simulink model "dcmtrCtrl_PID_Harness0"  (R2021a)
settings: Solver=ode15s  StartTime=0.0  StopTime=25  RelTol=1e-3
libraries: simulink_extras x2
settings Model: DataDictionary=dcmtr_ctrl.sldd  Creator=smuckati  LastModifiedBy=smuckati
settings OptimizationCC: DefaultParameterBehavior=Inlined  UseDivisionForNetSlopeComputation=on  EnhancedBackFolding=on  PassReuseOutputArgsAs=Individual arguments  ZeroExternalMemoryAtStartup=off  ZeroInternalMemoryAtStartup=off  OptimizeBlockOrder=speed  DifferentSizesBufferReuse=on  OptimizationCustomize=off  EfficientTunableParamExpr=on
settings DebuggingCC: SignalRangeChecking=error  ParameterPrecisionLossMsg=none  ParameterTunabilityLossMsg=error
settings SFSimCC: MATLABDynamicMemAlloc=off
settings RTWCC: SystemTargetFile=ert.tlc  GenCodeOnly=on  TemplateMakefile=ert_default_tmf  CodeExecutionProfiling=on  CodeProfilingSaveOptions=AllData  CodeProfilingInstrumentation=detailed
settings CodeAppCC: ForceParamTrailComments=on  IgnoreCustomStorageClasses=off  OperatorAnnotations=on  SimulinkDataObjDesc=on  SFDataObjDesc=on  InsertBlockDesc=on
settings ERTTargetCC: TargetLangStandard=C99 (ISO)  GenerateSampleERTMain=on  InlinedParameterPlacement=NonHierarchical  ERTCustomFileTemplate=example_file_process.tlc

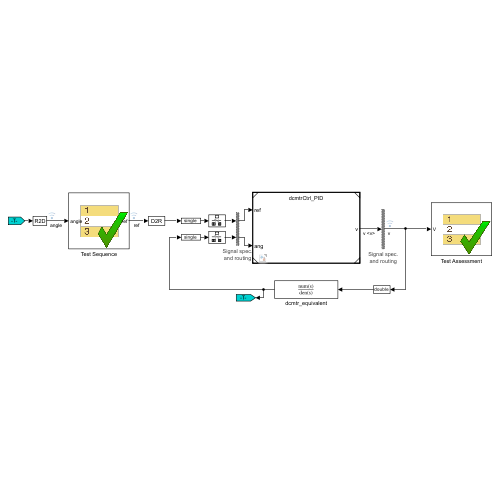
[thumbnail: Simulink's stored preview of the top-level diagram]
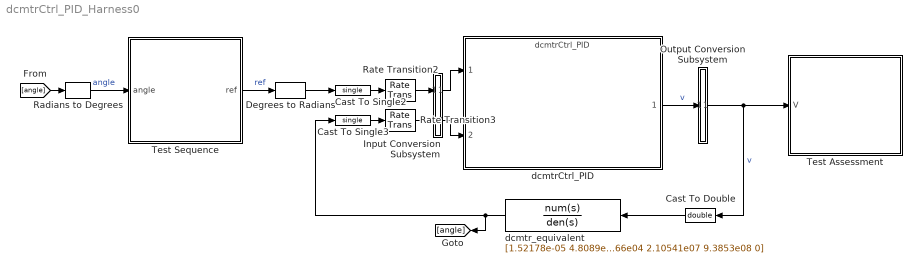
== system dcmtrCtrl_PID_Harness0 ==
  Cast To Double : DataTypeConversion  OutDataTypeStr=double
  Cast To Single2 : DataTypeConversion  OutDataTypeStr=single
  Cast To Single3 : DataTypeConversion  OutDataTypeStr=single
  Degrees to Radians : simulink_extras/Transformations/Degrees to Radians
  Input Conversion Subsystem : Subsystem  Tag=__SLT_ICS__  Description=|
      | Signal spec.
      | and routing
      settings: AttributesFormatString=%<Description>
  Output Conversion Subsystem : Subsystem  Tag=__SLT_OCS__  Description=|
      | Signal spec.
      | and routing
      settings: AttributesFormatString=%<Description>
  Radians to Degrees : simulink_extras/Transformations/Radians to Degrees
  Rate Transition2 : RateTransition  OutPortSampleTime=Ctrl_Ts
  Rate Transition3 : RateTransition  OutPortSampleTime=Ctrl_Ts
  Test Assessment : Test Sequence  TreatAsAtomicUnit=on
  Test Sequence : Test Sequence  TreatAsAtomicUnit=on
  dcmtrCtrl_PID : ModelReference  ModelNameDialog=dcmtrCtrl_PID  SimulationMode=Normal  ModelReferenceVersion=6.0
  dcmtr_equivalent : TransferFcn  Numerator=[1.52178e-05 4.8089e07]  Denominator=[1 1.74166e04 2.10541e07 9.3853e08 0]
  wires:
  Degrees to Radians/1 -> Cast To Single2/1
  Output Conversion Subsystem/1(Outport_1) -> Cast To Double/1, Test Assessment/1(V)  "v"
  Input Conversion Subsystem/1(Outport_1) -> dcmtrCtrl_PID/1
  Input Conversion Subsystem/2(Outport_2) -> dcmtrCtrl_PID/2
  dcmtrCtrl_PID/1 -> Output Conversion Subsystem/1(Inport_1)  "v"
  Cast To Single2/1 -> Rate Transition2/1
  Rate Transition2/1 -> Input Conversion Subsystem/1(Inport_1)
  Cast To Single3/1 -> Rate Transition3/1
  Rate Transition3/1 -> Input Conversion Subsystem/2(Inport_2)
  dcmtr_equivalent/1 -> [angle], Cast To Single3/1
  Cast To Double/1 -> dcmtr_equivalent/1
  Test Sequence/1(ref) -> Degrees to Radians/1  "ref"
  [angle] -> Radians to Degrees/1
  Radians to Degrees/1 -> Test Sequence/1(angle)  "angle"

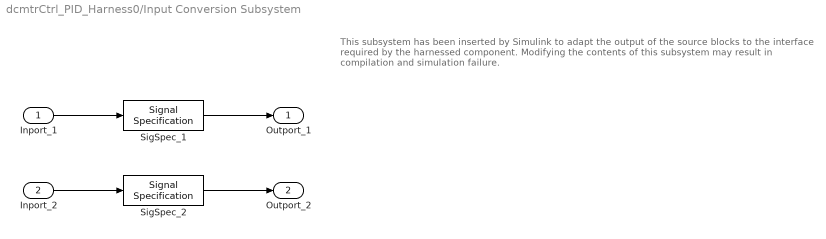
== system dcmtrCtrl_PID_Harness0/Input Conversion Subsystem ==
  note: This subsystem has been inserted by Simulink to adapt the output of the source blocks to the interface required by the harnessed component.
      |  Modifying the contents of this subsystem may result in compilation and simulation failure.
  Inport_1 : Inport
  Inport_2 : Inport  Port=2
  SigSpec_1 : SignalSpecification  OutDataTypeStr=single  Dimensions=[1]  SampleTime=0.01
  SigSpec_2 : SignalSpecification  OutDataTypeStr=single  Dimensions=[1]  SampleTime=0.01
  Outport_1 : Outport
  Outport_2 : Outport  Port=2
  wires:
  SigSpec_1/1 -> Outport_1/1
  Inport_1/1 -> SigSpec_1/1
  SigSpec_2/1 -> Outport_2/1
  Inport_2/1 -> SigSpec_2/1

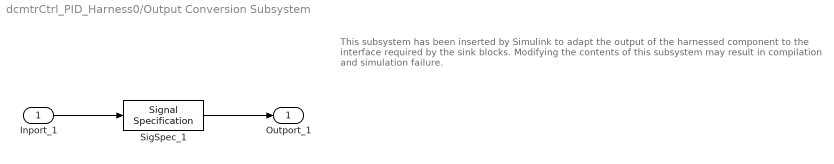
== system dcmtrCtrl_PID_Harness0/Output Conversion Subsystem ==
  note: This subsystem has been inserted by Simulink to adapt the output of the harnessed component to the interface required by the sink blocks.
      |  Modifying the contents of this subsystem may result in compilation and simulation failure.
  Inport_1 : Inport
  SigSpec_1 : SignalSpecification  OutDataTypeStr=single  Dimensions=[1]  SampleTime=0.01
  Outport_1 : Outport
  wires:
  Inport_1/1 -> SigSpec_1/1
  SigSpec_1/1 -> Outport_1/1

== stateflow chart dcmtrCtrl_PID_Harness0/Test Assessment ==
  state MOTOR_REST
  state MONITOR_MAX_VOLT
    verify( abs(V) <= 5);
  (default) -> MOTOR_REST
  MOTOR_REST -> MONITOR_MAX_VOLT : [
      | after(1,sec)
      | ]
  data: V input

== stateflow chart dcmtrCtrl_PID_Harness0/Test Sequence ==
  state MOTOR_INITIALIZE
    ref = 0;
  state STEP_UP
    ref = 20;
  state CHECK_SETTLE
    ref = 20;
  state MOTOR_DEFAULT
    ref = 0;
  state SMOOTH_SINE
    ref = 20*sin(et*2*pi/20);
    state SMOOTH_SINE_1
    (default) -> SMOOTH_SINE_1
  (default) -> MOTOR_INITIALIZE
  MOTOR_INITIALIZE -> STEP_UP : [
      | after(1,sec)
      | ]
  STEP_UP -> CHECK_SETTLE : [
      | after(3,sec)
      | ]
  CHECK_SETTLE -> MOTOR_DEFAULT : [
      | (angle - ref) < 0.20
      | ]
  MOTOR_DEFAULT -> SMOOTH_SINE : [
      | after(5,sec)
      | ]
  SMOOTH_SINE -> MOTOR_DEFAULT : [
      | angle < -5
      | ]
  data: ref output; angle input
